simulink model "model2"  (R2019b)
settings: Solver=VariableStepAuto  StartTime=0.0  StopTime=50  RelTol=1e-3
values from neighbouring files (symbols this model uses):
  gamma1 = 4    [odev3.m]
  gamma2 = 0.2    [odev3.m]
settings Model: Creator=Mustafa Sezer  LastModifiedBy=Mustafa Sezer

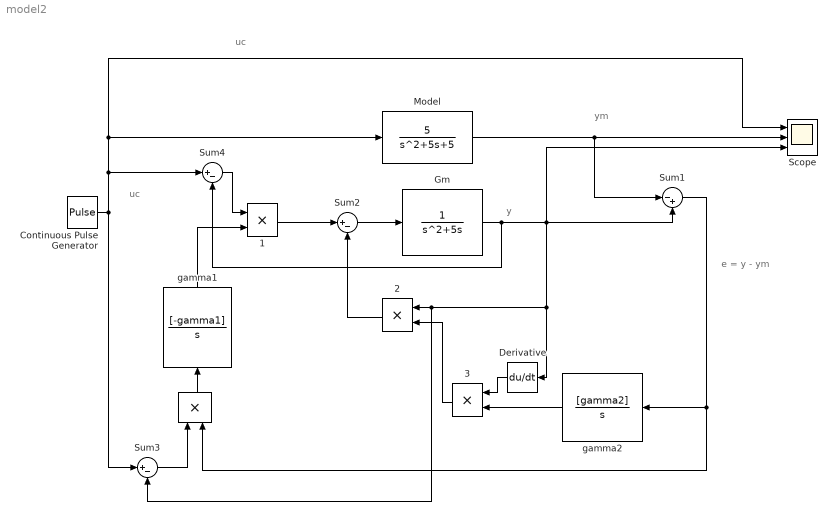
== system model2 ==
  note: uc
  note: uc
  note: y
  note: e = y - ym
  note: ym
   {,1..3} (4 alike) : Product
  Continuous Pulse Generator : DiscretePulseGenerator  PulseType=Time based  Period=20  PulseWidth=50
  Derivative : Derivative
  "Gm  " : TransferFcn  Denominator=[1 5 0]
  Model : TransferFcn  Numerator=[5]  Denominator=[1 5 5]
  Scope : Scope  NumInputPorts=3
  Sum1 : Sum  Inputs=|-+
  Sum2 : Sum  Inputs=|+-
  Sum3 : Sum  Inputs=|+-
  Sum4 : Sum  Inputs=|+-
  "gamma1 " : TransferFcn  Numerator=[-gamma1]  Denominator=[1 0]
  gamma2 : TransferFcn  Numerator=[gamma2]  Denominator=[1 0]
  wires:
  gamma2/1 -> " 3"/2
  " 3"/1 -> " 2"/2
  " 2"/1 -> Sum2/2
  Sum2/1 -> "Gm  "/1
  " 1"/1 -> Sum2/1
  "gamma1 "/1 -> " 1"/2
  Model/1 -> Scope/2, Sum1/1
  Continuous Pulse Generator/1 -> Sum4/1, Model/1, Scope/1, Sum3/1
  "Gm  "/1 -> Sum4/2, Derivative/1, Sum3/2, " 2"/1, Scope/3, Sum1/2
  Sum1/1 -> gamma2/1, " "/2
  " "/1 -> "gamma1 "/1
  Sum3/1 -> " "/1
  Derivative/1 -> " 3"/1
  Sum4/1 -> " 1"/1
